simulink model "Cognata_Amp_split"  (R2022b)
settings: Solver=VariableStepAuto  StartTime=0.0  StopTime=inf  RelTol=1e-3
StopFcn:
  | pub_ros
model workspace (MAT data in the model file):
  WinSize = Simulink.Parameter
  WinSize.Value = 16
  WinSize.DataType = 'double'
  WinSize.Complexity = 'real'
  WinSize.Dimensions = [1 1]
  fc_bandpass = Simulink.Parameter
  fc_bandpass.Value = [0.05 0.26]
  fc_bandpass.DataType = 'double'
  fc_bandpass.Complexity = 'real'
  fc_bandpass.Dimensions = [1 2]
libraries: robotlib x3, dspnetwork x1
settings Model: Creator=music  LastModifiedBy=LAB-OREN1

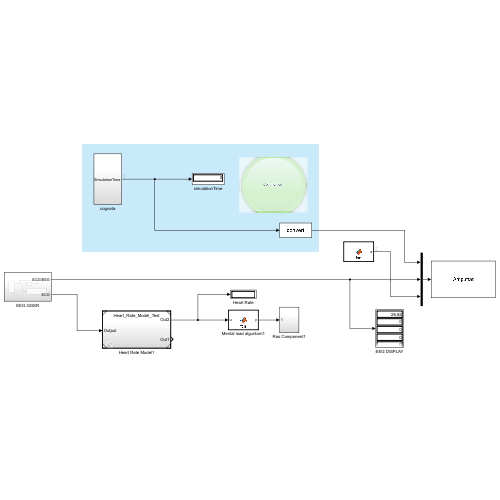
[thumbnail: Simulink's stored preview of the top-level diagram]
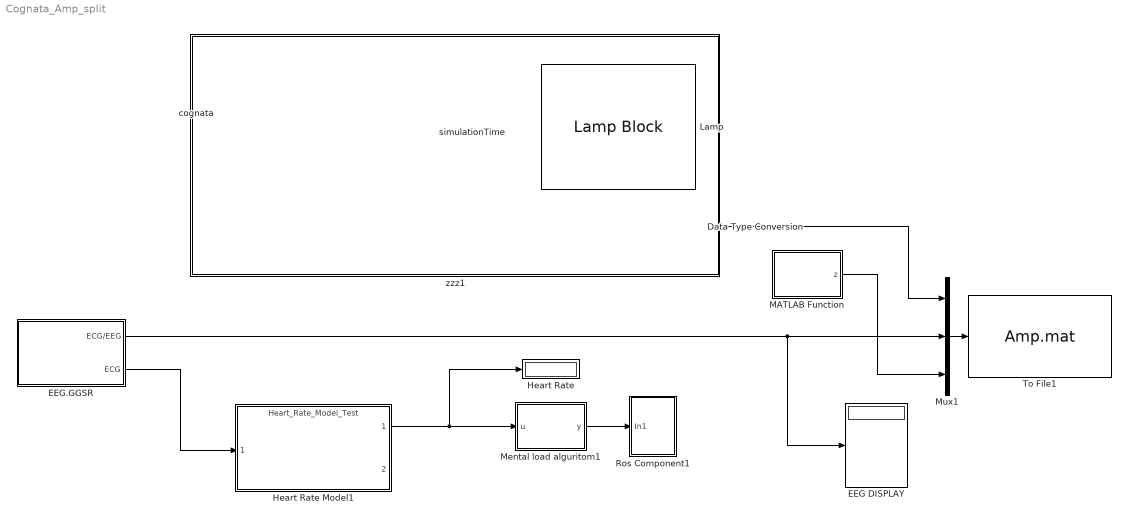
== system Cognata_Amp_split ==
  Data Type Conversion : DataTypeConversion  SaturateOnIntegerOverflow=off  RndMeth=Floor
  EEG DISPLAY : Display
  EEG.GGSR : Subsystem
  Heart Rate : Display
  Heart Rate Model1 : ModelReference  ModelNameDialog=Heart_Rate_Model_Test  SimulationMode=Normal  ModelReferenceVersion=2.18.00
  Lamp : LampBlock
  MATLAB Function : MATLAB Function  TreatAsAtomicUnit=on
  Mental load alguritom1 : MATLAB Function  TreatAsAtomicUnit=on
  Mux1 : Mux  Inputs=3
  Ros Component1 : Subsystem
  To File1 : ToFile  Filename=Amp.mat  MatrixName=Ampdata  SampleTime=0.008
  cognata : Subsystem
  simulationTime : Display
  zzz1 : Subsystem  TreatAsAtomicUnit=on
      settings: OpenFcn=% no-op
      mask Display: disp('')
  wires:
  Mux1/1 -> To File1/1
  Data Type Conversion/1 -> Mux1/1
  MATLAB Function/1(z) -> Mux1/3
  cognata/1(SimulationTime) -> simulationTime/1, Data Type Conversion/1
  EEG.GGSR/1(ECG/EEG) -> EEG DISPLAY/1, Mux1/2
  Heart Rate Model1/1 -> Mental load alguritom1/1(u), Heart Rate/1
  Mental load alguritom1/1(y) -> Ros Component1/1(In1)
  EEG.GGSR/2(ECG) -> Heart Rate Model1/1

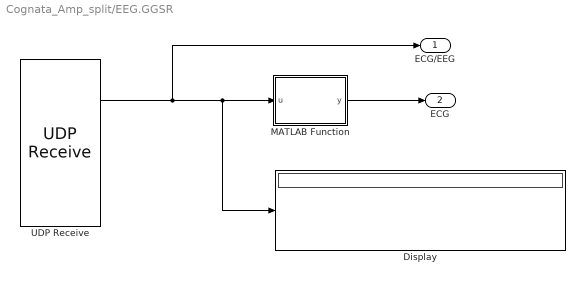
== system Cognata_Amp_split/EEG.GGSR ==
  Display : Display
  MATLAB Function : MATLAB Function  TreatAsAtomicUnit=on
  UDP Receive : dspnetwork/UDP Receive  localURL='0.0.0.0'  localPort=49004  remoteURL='127.0.0.1'  remotePort=-1  recvBufferSize=41  dims=13  signalDatatype=double  isComplex=off  isVarSize=off  showBlockingTime=off  blockingTime=0  sampletime=0.008  blockPlatform=[]
  ECG/EEG : Outport
  ECG : Outport  Port=2
  wires:
  UDP Receive/1 -> ECG/EEG/1, Display/1, MATLAB Function/1(u)
  MATLAB Function/1(y) -> ECG/1

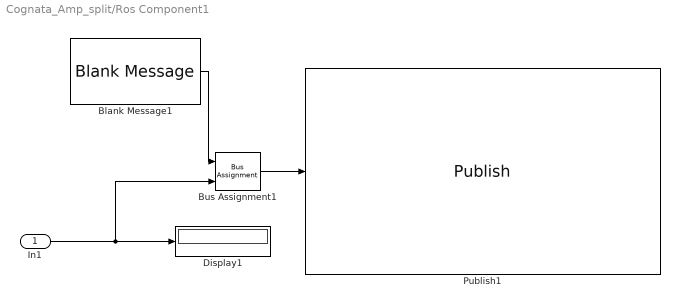
== system Cognata_Amp_split/Ros Component1 ==
  In1 : Inport
  Blank Message1 : robotlib/Blank Message  messageClass=Message  entityType=std_msgs/Float64  messageType=std_msgs/Float64  SampleTime=inf  legacyBusStruct=off
  Bus Assignment1 : BusAssignment  AssignedSignals=Data
  Display1 : Display
  Publish1 : robotlib/Publish  topicSource=Specify your own  topic=/HR  messageType=std_msgs/Float64  legacyBusStruct=off  messageQueueLength=1
  wires:
  In1/1 -> Bus Assignment1/2, Display1/1
  Bus Assignment1/1 -> Publish1/1
  Blank Message1/1 -> Bus Assignment1/1

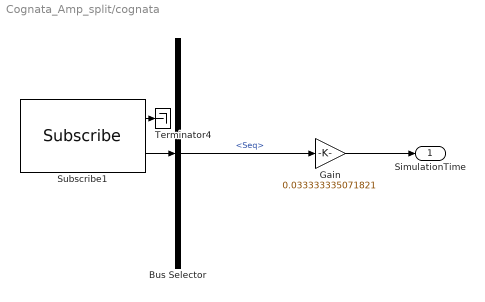
== system Cognata_Amp_split/cognata ==
  Bus Selector : BusSelector  OutputSignals=Header.Seq
  Gain : Gain  Gain=0.033333335071821
  Subscribe1 : robotlib/Subscribe  topicSource=Specify your own  topic=/cognataSDK/GPS/info  messageType=sensor_msgs/NavSatFix  SampleTime=0.001953125  legacyBusStruct=off  messageQueueLength=10
  Terminator4 : Terminator
  SimulationTime : Outport
  wires:
  Bus Selector/1 -> Gain/1  "<Seq>"
  Subscribe1/2 -> Bus Selector/1
  Gain/1 -> SimulationTime/1
  Subscribe1/1 -> Terminator4/1

== system Cognata_Amp_split/zzz1 ==

== matlab function Cognata_Amp_split/MATLAB Function ==
  data: z output
function z = fcn()
eml.extrinsic('clock'); 
t = [0,0,0,0,0,0];
t = clock;
k = t(1,4:6);
z = k';
end

== matlab function Cognata_Amp_split/Mental load alguritom1 ==
  data: u input; y output
function y = fcn(u)

y= probability_of_mental_howrkload(u);

end

== matlab function Cognata_Amp_split/EEG.GGSR/MATLAB Function ==
  data: u input; y output
function y = fcn(u)

y = u(1);
